simulink model "TestTurbine"  (R2012b)
settings: Solver=ode45  StartTime=0.0  StopTime=10.0  RelTol=1e-3
settings Model: Creator=tlavelle  LastModifiedBy=tlavelle

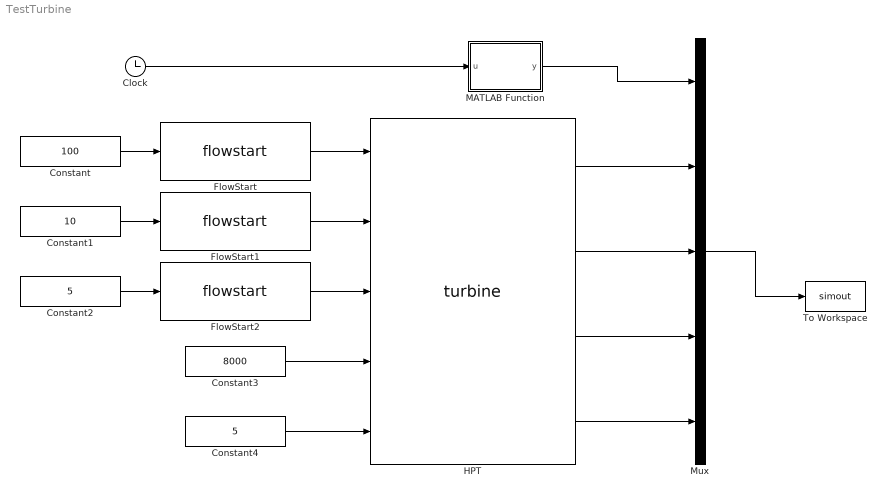
== system TestTurbine ==
  Clock : Clock
  Constant : Constant  Value=100
  Constant1 : Constant  Value=10
  Constant2 : Constant  Value=5
  Constant3 : Constant  Value=8000
  Constant4 : Constant  Value=5
  FlowStart : M-S-Function  FunctionName=flowstart  Parameters=Tt,Pt,comp1,comp2,comp3,comp4,comp5,comp6  mask{Tt=2500, Pt=297.127, comp1=1, comp2=0, comp3=.025, comp4=0, comp5=0, comp6=0}
      mask prompts: Tt "Exit Temperature"; Pt "Exit Pressure"
      mask Display:
      | color('red'); port_label('input',1,'Flow')
      | color('red'); port_label('output',1,'Flow Out')
  FlowStart1 : M-S-Function  FunctionName=flowstart  Parameters=Tt,Pt,comp1,comp2,comp3,comp4,comp5,comp6  mask{Tt=1398, Pt=297.127, comp1=1, comp2=0, comp3=0, comp4=0, comp5=0, comp6=0}
      mask prompts: Tt "Exit Temperature"; Pt "Exit Pressure"
      mask Display:
      | color('red'); port_label('input',1,'Flow')
      | color('red'); port_label('output',1,'Flow Out')
  FlowStart2 : M-S-Function  FunctionName=flowstart  Parameters=Tt,Pt,comp1,comp2,comp3,comp4,comp5,comp6  mask{Tt=1398, Pt=297.127, comp1=1, comp2=0, comp3=0, comp4=0, comp5=0, comp6=0}
      mask prompts: Tt "Exit Temperature"; Pt "Exit Pressure"
      mask Display:
      | color('red'); port_label('input',1,'Flow')
      | color('red'); port_label('output',1,'Flow Out')
  HPT : M-S-Function  FunctionName=turbine  Parameters=MapFile,NcDes,effDes,PRmapDes,Ndes,BSW1,BSW2,s_eff,s_Wc,s_C_Nc,s_PR,IDes  mask{MapFile='HPT1.map', NcDes=100, effDes=.913, PRmapDes=4.9299, Ndes=7499, BSW1=1, BSW2=0, s_eff=0, s_Wc=0, s_C_Nc=0, s_PR=0, IDes=0}
      mask prompts: MapFile "Map File"; NcDes "Design Speed"; effDes "Design efficiency"; PRmapDes "Design Pressure Ratio Map"; Ndes "N des"; BSW1 "Bleed 1 Switch (1 front 0 back)"; BSW2 "Bleed 2 Swtich (1 front 0 back )"; s_eff "Input map efficiency scalar"; s_Wc "Input map correct weight flow scala"; s_C_Nc "Input map speed scalar"; s_PR "Input map pressure ratio scalar"
      mask Display:
      | color('blue'); port_label('input',1,'Flow In')
      | color('blue'); port_label('input',2,'Bleed 1')
      | color('blue'); port_label('input',3,'Bleed 2')
      | color('red'); port_label('input',4,'Speed')
      | color('darkgreen'); port_label('input',5,'PR')
      | 
      | color('blue'); port_label('output',1,'Flow Out')
      | color('green'); port_label('output',2,'Flow Error')
      | color('black'); port_label('output',3,'Power')
  MATLAB Function : MATLAB Function  TreatAsAtomicUnit=on
  Mux : Mux  Inputs=5
  To Workspace : ToWorkspace  VariableName=simout  SampleTime=-1  SaveFormat=Timeseries
  wires:
  Constant2/1 -> FlowStart2/1
  Constant1/1 -> FlowStart1/1
  Constant/1 -> FlowStart/1
  FlowStart/1 -> HPT/1
  FlowStart1/1 -> HPT/2
  FlowStart2/1 -> HPT/3
  Constant3/1 -> HPT/4
  Constant4/1 -> HPT/5
  Mux/1 -> To Workspace/1
  Clock/1 -> MATLAB Function/1(u)
  MATLAB Function/1(y) -> Mux/1
  HPT/1 -> Mux/2
  HPT/2 -> Mux/3
  HPT/3 -> Mux/4
  HPT/4 -> Mux/5

== matlab function TestTurbine/MATLAB Function ==
  data: u input; y output
function y = fcn(u)
%#codegen
eml.extrinsic('set_param');
if u < 3
   set_param('TestTurbine/HPT','IDes','0');
elseif u< 6 
   set_param('TestTurbine/HPT','IDes','1'); 
else 
   set_param('TestTurbine/HPT','IDes','2'); 
end    
y = u;
